simulink model "Online_Ordering_System_Activity_Diagram"  (R2024a)
settings: Solver=VariableStepAuto  StartTime=0.0  StopTime=10.0  RelTol=1e-3
(part 1 of 2)
settings Model: Creator=OdaNobuyuki  LastModifiedBy=OdaNobuyuki

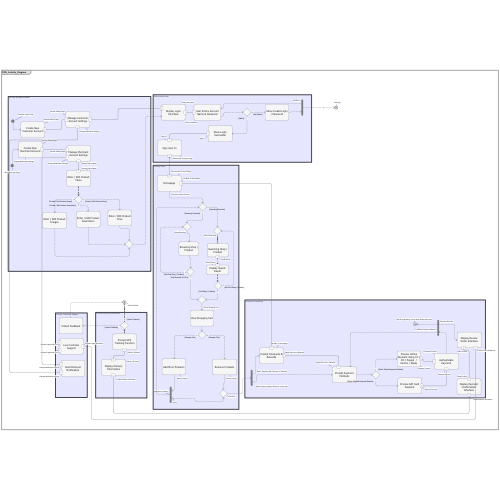
[thumbnail: Simulink's stored preview of the top-level diagram]
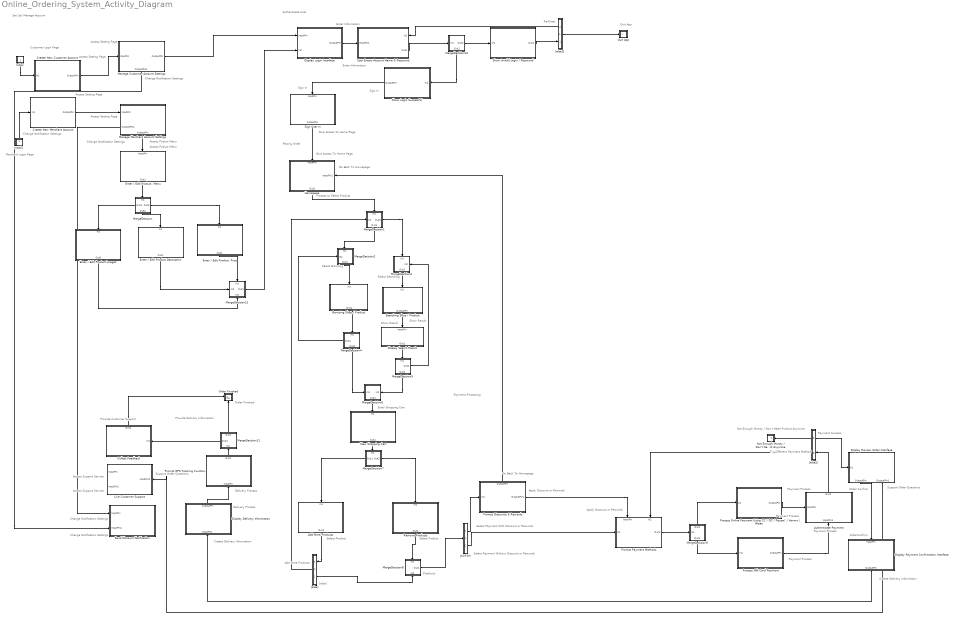
== system Online_Ordering_System_Activity_Diagram ==
  note: Support Order Questions
  note: Access Setting Page
  note: Re-Enter
  note: Enter Information
  note: Enter Information
  note: Give Access To Home Page
  note: Give Access To Home Page
  note: Show Result
  note: Show Result
  note: Access Support Service
  note: Change Notification Settings
  note: Change Notification Settings
  note: Change Notification Settings
  note: Provide Customer Support
  note: Merchant Login Page
  note: Customer Login Page
  note: Set Up/ Manage Account
  note: Delivery Process
  note: Delivery Process
  note: Create Delivery Information
  note: Create Delivery Information
  note: OrderConfirm
  note: Order Confirm
  note: Payment Success
  note: Try Different Payment Method
  note: Payment Process
  note: Payment Process
  note: Order Finished
  note: Quit App
  note: Not Enough Money / Don't Need Product Anymore
  note: Go Back To Homepage
  note: Apply Discount or Rewords
  note: Select Payment With Discount or Rewords
  note: Select Payment Without Discount or Rewords
  note: Enter Shopping Cart
  note: Add More Products
  note: Checkout
  note: [else]
  note: Select Product
  note: Select Product
  note: Select Searching
  note: Select Browsing
  note: Process to Select Product
  note: Sign In
  note: Provide Delivery Information
  note: Payment Processing
  note: Placing Order
  note: Authenticate User
  note: Access Setting Page
  note: Access Setting Page
  note: Access Setting Page
  note: Access Poduct Menu
  note: Access Poduct Menu
  note: Go Back To Homepage
  note: Apply Discount or Rewords
  note: Payment Process
  note: Payment Process
  note: Sign In
  note: Access Support Service
  note: Change Notification Settings
  note: Change Notification Settings
  note: Support Order Questions
  Add More Products : Subsystem
      settings: CopyFcn=set_param(gcbh,'LinkStatus','none');  PortSchema="{\"entries\":[{\"content\":{\"sides\":[{\"content\":{},\"type\":\"ConnectorPlacement.EquallySpacedRectSide\",\"uuid\":\"bfcd81ca-6cc0-42fb-99a3-45b9e2418847\"},{\"content\":{\"side\":\"RIGHT\"},\"type\":\"ConnectorPlacement.EquallySpacedRectSide\",\"uuid\":\"2a8794f4-3879-4bca-94c5-223b002e6000\"},{\"content\":{\"connectorIds\":[\"In1\"],\"side\":\"TOP\"},\"type\":\"ConnectorPlacement.EquallySpacedRectSide\",\"uuid\":\"3a486ab2-570b-44bd-b64c-1f33147c21a8\"},{\"content\":{\"connectorIds\":[\"Out1\"],\"side\":\"BOTTOM\"},\"type\":\"ConnectorPlacement.EquallySpacedRectSide\",\"uuid\":\"d015d86f-4011-41b5-baf2-3a54511849a1\"}]},\"type\":\"ConnectorPlacement.EquallySpacedConnector\",\"uuid\":\"4fcb30da-47fd-4892-8b00-93a0afe24f69\"}],\"packageUris\":[\"http://schema.mathworks.com/mf0/Connector/R2020b\"],\"version\":\"1.0\"}"
  Authenticate Payment : Subsystem
      settings: CopyFcn=set_param(gcbh,'LinkStatus','none');  PortSchema="{\"entries\":[{\"content\":{\"sides\":[{\"content\":{\"connectorIds\":[\"In1\"]},\"type\":\"ConnectorPlacement.EquallySpacedRectSide\",\"uuid\":\"be42d590-71f1-4328-bf36-769bf487d98c\"},{\"content\":{\"side\":\"RIGHT\"},\"type\":\"ConnectorPlacement.EquallySpacedRectSide\",\"uuid\":\"f686bdea-c754-42dd-9eaf-f93e30a31542\"},{\"content\":{\"connectorIds\":[\"Out1\"],\"side\":\"TOP\"},\"type\":\"ConnectorPlacement.EquallySpacedRectSide\",\"uuid\":\"aaf7fed9-1a14-44f9-b7af-ebaa0b7204d4\"},{\"content\":{\"connectorIds\":[\"In2\"],\"side\":\"BOTTOM\"},\"type\":\"ConnectorPlacement.EquallySpacedRectSide\",\"uuid\":\"9a6b8873-b7d5-47b2-be69-ed4b1ca685af\"}]},\"type\":\"ConnectorPlacement.EquallySpacedConnector\",\"uuid\":\"f2ca7d40-436a-4bcc-bce4-1a0ffaec5aa3\"}],\"packageUris\":[\"http://schema.mathworks.com/mf0/Connector/R2020b\"],\"version\":\"1.0\"}"
  Browsing Shop / Product : Subsystem
      settings: CopyFcn=set_param(gcbh,'LinkStatus','none');  PortSchema="{\"entries\":[{\"content\":{\"sides\":[{\"content\":{},\"type\":\"ConnectorPlacement.EquallySpacedRectSide\",\"uuid\":\"bfcd81ca-6cc0-42fb-99a3-45b9e2418847\"},{\"content\":{\"side\":\"RIGHT\"},\"type\":\"ConnectorPlacement.EquallySpacedRectSide\",\"uuid\":\"2a8794f4-3879-4bca-94c5-223b002e6000\"},{\"content\":{\"connectorIds\":[\"In1\"],\"side\":\"TOP\"},\"type\":\"ConnectorPlacement.EquallySpacedRectSide\",\"uuid\":\"3a486ab2-570b-44bd-b64c-1f33147c21a8\"},{\"content\":{\"connectorIds\":[\"Out1\"],\"side\":\"BOTTOM\"},\"type\":\"ConnectorPlacement.EquallySpacedRectSide\",\"uuid\":\"3ce360b7-2dac-440f-b63d-3367f7e15e3d\"}]},\"type\":\"ConnectorPlacement.EquallySpacedConnector\",\"uuid\":\"4fcb30da-47fd-4892-8b00-93a0afe24f69\"}],\"packageUris\":[\"http://schema.mathworks.com/mf0/Connector/R2020b\"],\"version\":\"1.0\"}"
  Collect Feedback : Subsystem
      settings: CopyFcn=set_param(gcbh,'LinkStatus','none');  PortSchema="{\"entries\":[{\"content\":{\"sides\":[{\"content\":{},\"type\":\"ConnectorPlacement.EquallySpacedRectSide\",\"uuid\":\"bfcd81ca-6cc0-42fb-99a3-45b9e2418847\"},{\"content\":{\"connectorIds\":[\"In1\"],\"side\":\"RIGHT\"},\"type\":\"ConnectorPlacement.EquallySpacedRectSide\",\"uuid\":\"2a8794f4-3879-4bca-94c5-223b002e6000\"},{\"content\":{\"connectorIds\":[\"Out1\"],\"side\":\"TOP\"},\"type\":\"ConnectorPlacement.EquallySpacedRectSide\",\"uuid\":\"3a486ab2-570b-44bd-b64c-1f33147c21a8\"}]},\"type\":\"ConnectorPlacement.EquallySpacedConnector\",\"uuid\":\"4fcb30da-47fd-4892-8b00-93a0afe24f69\"}],\"packageUris\":[\"http://schema.mathworks.com/mf0/Connector/R2020b\"],\"version\":\"1.0\"}"
  Create New Customer Account : Subsystem
      settings: CopyFcn=set_param(gcbh,'LinkStatus','none');
  Create New Merchant Account : Subsystem
      settings: CopyFcn=set_param(gcbh,'LinkStatus','none');
  Display Delivery Information : Subsystem
      settings: CopyFcn=set_param(gcbh,'LinkStatus','none');  PortSchema="{\"entries\":[{\"content\":{\"sides\":[{\"content\":{},\"type\":\"ConnectorPlacement.EquallySpacedRectSide\",\"uuid\":\"bfcd81ca-6cc0-42fb-99a3-45b9e2418847\"},{\"content\":{\"side\":\"RIGHT\"},\"type\":\"ConnectorPlacement.EquallySpacedRectSide\",\"uuid\":\"2a8794f4-3879-4bca-94c5-223b002e6000\"},{\"content\":{\"connectorIds\":[\"Out1\"],\"side\":\"TOP\"},\"type\":\"ConnectorPlacement.EquallySpacedRectSide\",\"uuid\":\"3a486ab2-570b-44bd-b64c-1f33147c21a8\"},{\"content\":{\"connectorIds\":[\"In1\"],\"side\":\"BOTTOM\"},\"type\":\"ConnectorPlacement.EquallySpacedRectSide\",\"uuid\":\"451f827c-7812-4a2b-baad-6237ef8a6df4\"}]},\"type\":\"ConnectorPlacement.EquallySpacedConnector\",\"uuid\":\"4fcb30da-47fd-4892-8b00-93a0afe24f69\"}],\"packageUris\":[\"http://schema.mathworks.com/mf0/Connector/R2020b\"],\"version\":\"1.0\"}"
  Display Login Interface : Subsystem
      settings: CopyFcn=set_param(gcbh,'LinkStatus','none');
  Display Payment Confirmation Interface : Subsystem
      settings: CopyFcn=set_param(gcbh,'LinkStatus','none');  PortSchema="{\"entries\":[{\"content\":{\"sides\":[{\"content\":{},\"type\":\"ConnectorPlacement.EquallySpacedRectSide\",\"uuid\":\"bfcd81ca-6cc0-42fb-99a3-45b9e2418847\"},{\"content\":{\"side\":\"RIGHT\"},\"type\":\"ConnectorPlacement.EquallySpacedRectSide\",\"uuid\":\"2a8794f4-3879-4bca-94c5-223b002e6000\"},{\"content\":{\"connectorIds\":[\"In1\"],\"side\":\"TOP\"},\"type\":\"ConnectorPlacement.EquallySpacedRectSide\",\"uuid\":\"3a486ab2-570b-44bd-b64c-1f33147c21a8\"},{\"content\":{\"connectorIds\":[\"Out1\"],\"side\":\"BOTTOM\"},\"type\":\"ConnectorPlacement.EquallySpacedRectSide\",\"uuid\":\"28139759-3bfc-43e8-9d7e-66a3114bf665\"}]},\"type\":\"ConnectorPlacement.EquallySpacedConnector\",\"uuid\":\"4fcb30da-47fd-4892-8b00-93a0afe24f69\"}],\"packageUris\":[\"http://schema.mathworks.com/mf0/Connector/R2020b\"],\"version\":\"1.0\"}"
  Display Review Order Interface : Subsystem
      settings: CopyFcn=set_param(gcbh,'LinkStatus','none');  PortSchema="{\"entries\":[{\"content\":{\"sides\":[{\"content\":{\"connectorIds\":[\"In1\"]},\"type\":\"ConnectorPlacement.EquallySpacedRectSide\",\"uuid\":\"6471ad79-39b4-4759-a736-ca09eeb8c1bf\"},{\"content\":{\"side\":\"RIGHT\"},\"type\":\"ConnectorPlacement.EquallySpacedRectSide\",\"uuid\":\"577ddd5b-f3b1-45a9-9feb-d7da88de3d28\"},{\"content\":{\"side\":\"TOP\"},\"type\":\"ConnectorPlacement.EquallySpacedRectSide\",\"uuid\":\"a229a248-5801-42c4-bc3a-df671f0dafbe\"},{\"content\":{\"connectorIds\":[\"Out1\",\"Out2\"],\"side\":\"BOTTOM\"},\"type\":\"ConnectorPlacement.EquallySpacedRectSide\",\"uuid\":\"31b6ee13-f671-41c4-9aa0-03afb235cf6a\"}]},\"type\":\"ConnectorPlacement.EquallySpacedConnector\",\"uuid\":\"7c76ea2b-17e6-4374-81ee-74665aad13d5\"}],\"packageUris\":[\"http://schema.mathworks.com/mf0/Connector/R2020b\"],\"version\":\"1.0\"}"
  Display Search Result : Subsystem
      settings: CopyFcn=set_param(gcbh,'LinkStatus','none');  PortSchema="{\"entries\":[{\"content\":{\"sides\":[{\"content\":{},\"type\":\"ConnectorPlacement.EquallySpacedRectSide\",\"uuid\":\"873ca6fb-737d-4b52-910b-d3362c79eeee\"},{\"content\":{\"side\":\"RIGHT\"},\"type\":\"ConnectorPlacement.EquallySpacedRectSide\",\"uuid\":\"ba60fc33-b236-4c23-8fcd-c0b31457fe6e\"},{\"content\":{\"connectorIds\":[\"In1\"],\"side\":\"TOP\"},\"type\":\"ConnectorPlacement.EquallySpacedRectSide\",\"uuid\":\"e81623ee-00f7-4aa0-b91b-b5c706a16c15\"},{\"content\":{\"connectorIds\":[\"Out1\"],\"side\":\"BOTTOM\"},\"type\":\"ConnectorPlacement.EquallySpacedRectSide\",\"uuid\":\"d2aa41e5-f0a2-4b95-961a-6292840acb60\"}]},\"type\":\"ConnectorPlacement.EquallySpacedConnector\",\"uuid\":\"4a5fb8e3-3bb7-4720-ba76-c4b22f03e2da\"}],\"packageUris\":[\"http://schema.mathworks.com/mf0/Connector/R2020b\"],\"version\":\"1.0\"}"
  Enter / Edit Product  Menu : Subsystem
      settings: CopyFcn=set_param(gcbh,'LinkStatus','none');  PortSchema="{\"entries\":[{\"content\":{\"sides\":[{\"content\":{},\"type\":\"ConnectorPlacement.EquallySpacedRectSide\",\"uuid\":\"873ca6fb-737d-4b52-910b-d3362c79eeee\"},{\"content\":{\"side\":\"RIGHT\"},\"type\":\"ConnectorPlacement.EquallySpacedRectSide\",\"uuid\":\"ba60fc33-b236-4c23-8fcd-c0b31457fe6e\"},{\"content\":{\"connectorIds\":[\"In1\"],\"side\":\"TOP\"},\"type\":\"ConnectorPlacement.EquallySpacedRectSide\",\"uuid\":\"e81623ee-00f7-4aa0-b91b-b5c706a16c15\"},{\"content\":{\"connectorIds\":[\"Out1\"],\"side\":\"BOTTOM\"},\"type\":\"ConnectorPlacement.EquallySpacedRectSide\",\"uuid\":\"f87e1b9f-2237-41b3-9347-c624be7169f3\"}]},\"type\":\"ConnectorPlacement.EquallySpacedConnector\",\"uuid\":\"4a5fb8e3-3bb7-4720-ba76-c4b22f03e2da\"}],\"packageUris\":[\"http://schema.mathworks.com/mf0/Connector/R2020b\"],\"version\":\"1.0\"}"
  Enter / Edit Product  Price : Subsystem
      settings: CopyFcn=set_param(gcbh,'LinkStatus','none');  PortSchema="{\"entries\":[{\"content\":{\"sides\":[{\"content\":{},\"type\":\"ConnectorPlacement.EquallySpacedRectSide\",\"uuid\":\"873ca6fb-737d-4b52-910b-d3362c79eeee\"},{\"content\":{\"side\":\"RIGHT\"},\"type\":\"ConnectorPlacement.EquallySpacedRectSide\",\"uuid\":\"ba60fc33-b236-4c23-8fcd-c0b31457fe6e\"},{\"content\":{\"connectorIds\":[\"In1\"],\"side\":\"TOP\"},\"type\":\"ConnectorPlacement.EquallySpacedRectSide\",\"uuid\":\"e81623ee-00f7-4aa0-b91b-b5c706a16c15\"},{\"content\":{\"connectorIds\":[\"Out1\"],\"side\":\"BOTTOM\"},\"type\":\"ConnectorPlacement.EquallySpacedRectSide\",\"uuid\":\"39b948d7-5fed-498d-a70d-5c860efeabd0\"}]},\"type\":\"ConnectorPlacement.EquallySpacedConnector\",\"uuid\":\"4a5fb8e3-3bb7-4720-ba76-c4b22f03e2da\"}],\"packageUris\":[\"http://schema.mathworks.com/mf0/Connector/R2020b\"],\"version\":\"1.0\"}"
  Enter / Edit Product Description : Subsystem
      settings: CopyFcn=set_param(gcbh,'LinkStatus','none');  PortSchema="{\"entries\":[{\"content\":{\"sides\":[{\"content\":{},\"type\":\"ConnectorPlacement.EquallySpacedRectSide\",\"uuid\":\"873ca6fb-737d-4b52-910b-d3362c79eeee\"},{\"content\":{\"side\":\"RIGHT\"},\"type\":\"ConnectorPlacement.EquallySpacedRectSide\",\"uuid\":\"ba60fc33-b236-4c23-8fcd-c0b31457fe6e\"},{\"content\":{\"connectorIds\":[\"In1\"],\"side\":\"TOP\"},\"type\":\"ConnectorPlacement.EquallySpacedRectSide\",\"uuid\":\"e81623ee-00f7-4aa0-b91b-b5c706a16c15\"},{\"content\":{\"connectorIds\":[\"Out1\"],\"side\":\"BOTTOM\"},\"type\":\"ConnectorPlacement.EquallySpacedRectSide\",\"uuid\":\"e9df8be3-2e0d-4814-bab8-e9195508b871\"}]},\"type\":\"ConnectorPlacement.EquallySpacedConnector\",\"uuid\":\"4a5fb8e3-3bb7-4720-ba76-c4b22f03e2da\"}],\"packageUris\":[\"http://schema.mathworks.com/mf0/Connector/R2020b\"],\"version\":\"1.0\"}"
  Enter / Edit Product Images : Subsystem
      settings: CopyFcn=set_param(gcbh,'LinkStatus','none');  PortSchema="{\"entries\":[{\"content\":{\"sides\":[{\"content\":{},\"type\":\"ConnectorPlacement.EquallySpacedRectSide\",\"uuid\":\"873ca6fb-737d-4b52-910b-d3362c79eeee\"},{\"content\":{\"side\":\"RIGHT\"},\"type\":\"ConnectorPlacement.EquallySpacedRectSide\",\"uuid\":\"ba60fc33-b236-4c23-8fcd-c0b31457fe6e\"},{\"content\":{\"connectorIds\":[\"In1\"],\"side\":\"TOP\"},\"type\":\"ConnectorPlacement.EquallySpacedRectSide\",\"uuid\":\"e81623ee-00f7-4aa0-b91b-b5c706a16c15\"},{\"content\":{\"connectorIds\":[\"Out1\"],\"side\":\"BOTTOM\"},\"type\":\"ConnectorPlacement.EquallySpacedRectSide\",\"uuid\":\"a34f8f4a-2331-4593-96e1-216def65723d\"}]},\"type\":\"ConnectorPlacement.EquallySpacedConnector\",\"uuid\":\"4a5fb8e3-3bb7-4720-ba76-c4b22f03e2da\"}],\"packageUris\":[\"http://schema.mathworks.com/mf0/Connector/R2020b\"],\"version\":\"1.0\"}"
  Homepage : Subsystem
      settings: CopyFcn=set_param(gcbh,'LinkStatus','none');  PortSchema="{\"entries\":[{\"content\":{\"sides\":[{\"content\":{},\"type\":\"ConnectorPlacement.EquallySpacedRectSide\",\"uuid\":\"9c7be66a-1772-4efc-8f14-7a500ca71a54\"},{\"content\":{\"connectorIds\":[\"In2\"],\"side\":\"RIGHT\"},\"type\":\"ConnectorPlacement.EquallySpacedRectSide\",\"uuid\":\"38f08e10-8633-45ed-b24d-07e293b2144f\"},{\"content\":{\"connectorIds\":[\"In1\"],\"side\":\"TOP\"},\"type\":\"ConnectorPlacement.EquallySpacedRectSide\",\"uuid\":\"9945d600-1a94-418c-9fd4-80c3bf52b6dd\"},{\"content\":{\"connectorIds\":[\"Out1\"],\"side\":\"BOTTOM\"},\"type\":\"ConnectorPlacement.EquallySpacedRectSide\",\"uuid\":\"639fe1aa-fc4f-4338-a28d-cf257359008e\"}]},\"type\":\"ConnectorPlacement.EquallySpacedConnector\",\"uuid\":\"f5f1796a-aeed-4e15-b522-4d9bae7d766e\"}],\"packageUris\":[\"http://schema.mathworks.com/mf0/Connector/R2020b\"],\"version\":\"1.0\"}"
  Initial : Subsystem
      settings: CopyFcn=set_param(gcbh,'LinkStatus','none');  PortSchema="{\"entries\":[{\"content\":{\"sides\":[{\"content\":{},\"type\":\"ConnectorPlacement.EquallySpacedRectSide\",\"uuid\":\"873ca6fb-737d-4b52-910b-d3362c79eeee\"},{\"content\":{\"side\":\"RIGHT\"},\"type\":\"ConnectorPlacement.EquallySpacedRectSide\",\"uuid\":\"ba60fc33-b236-4c23-8fcd-c0b31457fe6e\"},{\"content\":{\"side\":\"TOP\"},\"type\":\"ConnectorPlacement.EquallySpacedRectSide\",\"uuid\":\"e81623ee-00f7-4aa0-b91b-b5c706a16c15\"},{\"content\":{\"connectorIds\":[\"Out1\"],\"side\":\"BOTTOM\"},\"type\":\"ConnectorPlacement.EquallySpacedRectSide\",\"uuid\":\"754ea620-bcdd-4f6e-b1d6-7350cee697a7\"}]},\"type\":\"ConnectorPlacement.EquallySpacedConnector\",\"uuid\":\"4a5fb8e3-3bb7-4720-ba76-c4b22f03e2da\"}],\"packageUris\":[\"http://schema.mathworks.com/mf0/Connector/R2020b\"],\"version\":\"1.0\"}"
  Initial1 : Subsystem
      settings: CopyFcn=set_param(gcbh,'LinkStatus','none');  PortSchema="{\"entries\":[{\"content\":{\"sides\":[{\"content\":{},\"type\":\"ConnectorPlacement.EquallySpacedRectSide\",\"uuid\":\"873ca6fb-737d-4b52-910b-d3362c79eeee\"},{\"content\":{\"side\":\"RIGHT\"},\"type\":\"ConnectorPlacement.EquallySpacedRectSide\",\"uuid\":\"ba60fc33-b236-4c23-8fcd-c0b31457fe6e\"},{\"content\":{\"connectorIds\":[\"Out1\"],\"side\":\"TOP\"},\"type\":\"ConnectorPlacement.EquallySpacedRectSide\",\"uuid\":\"e81623ee-00f7-4aa0-b91b-b5c706a16c15\"}]},\"type\":\"ConnectorPlacement.EquallySpacedConnector\",\"uuid\":\"4a5fb8e3-3bb7-4720-ba76-c4b22f03e2da\"}],\"packageUris\":[\"http://schema.mathworks.com/mf0/Connector/R2020b\"],\"version\":\"1.0\"}"
  JoinFork : Subsystem
      settings: CopyFcn=set_param(gcbh,'LinkStatus','none');
  Live Customer Support : Subsystem
      settings: CopyFcn=set_param(gcbh,'LinkStatus','none');  PortSchema="{\"entries\":[{\"content\":{\"sides\":[{\"content\":{\"connectorIds\":[\"In1\",\"In2\"]},\"type\":\"ConnectorPlacement.EquallySpacedRectSide\",\"uuid\":\"5dac1142-e9ce-43d0-ba52-63279954a8b9\"},{\"content\":{\"connectorIds\":[\"In3\"],\"side\":\"RIGHT\"},\"type\":\"ConnectorPlacement.EquallySpacedRectSide\",\"uuid\":\"ca4fd33a-c89a-4006-bed6-b92bcf697d1b\"},{\"content\":{\"side\":\"TOP\"},\"type\":\"ConnectorPlacement.EquallySpacedRectSide\",\"uuid\":\"932f8a37-4771-496a-b31b-228ed95da92a\"}]},\"type\":\"ConnectorPlacement.EquallySpacedConnector\",\"uuid\":\"cf714b23-59d2-41ff-98fd-22561387faef\"}],\"packageUris\":[\"http://schema.mathworks.com/mf0/Connector/R2020b\"],\"version\":\"1.0\"}"
  Manage Customer Account Settings : Subsystem
      settings: CopyFcn=set_param(gcbh,'LinkStatus','none');  PortSchema="{\"entries\":[{\"content\":{\"sides\":[{\"content\":{\"connectorIds\":[\"In1\"]},\"type\":\"ConnectorPlacement.EquallySpacedRectSide\",\"uuid\":\"3fb5762c-1463-4d69-b71f-d3478a8e66fc\"},{\"content\":{\"connectorIds\":[\"Out1\"],\"side\":\"RIGHT\"},\"type\":\"ConnectorPlacement.EquallySpacedRectSide\",\"uuid\":\"8c5ab484-2882-4a25-a56e-8782928f7c87\"},{\"content\":{\"side\":\"TOP\"},\"type\":\"ConnectorPlacement.EquallySpacedRectSide\",\"uuid\":\"adc29f19-0a83-4db7-81d6-093442179a8b\"},{\"content\":{\"connectorIds\":[\"Out2\"],\"side\":\"BOTTOM\"},\"type\":\"ConnectorPlacement.EquallySpacedRectSide\",\"uuid\":\"551acee2-b4f2-469f-bccf-f435c30cc1a3\"}]},\"type\":\"ConnectorPlacement.EquallySpacedConnector\",\"uuid\":\"53417cf2-4b18-460a-8f45-b9110c6542e4\"}],\"packageUris\":[\"http://schema.mathworks.com/mf0/Connector/R2020b\"],\"version\":\"1.0\"}"
  Manage Merchant Account Settings : Subsystem
      settings: CopyFcn=set_param(gcbh,'LinkStatus','none');  PortSchema="{\"entries\":[{\"content\":{\"sides\":[{\"content\":{\"connectorIds\":[\"In1\",\"Out2\"]},\"type\":\"ConnectorPlacement.EquallySpacedRectSide\",\"uuid\":\"be42d590-71f1-4328-bf36-769bf487d98c\"},{\"content\":{\"side\":\"RIGHT\"},\"type\":\"ConnectorPlacement.EquallySpacedRectSide\",\"uuid\":\"f686bdea-c754-42dd-9eaf-f93e30a31542\"},{\"content\":{\"side\":\"TOP\"},\"type\":\"ConnectorPlacement.EquallySpacedRectSide\",\"uuid\":\"aaf7fed9-1a14-44f9-b7af-ebaa0b7204d4\"},{\"content\":{\"connectorIds\":[\"Out1\"],\"side\":\"BOTTOM\"},\"type\":\"ConnectorPlacement.EquallySpacedRectSide\",\"uuid\":\"0a28ab33-b43c-4e05-97e4-fa4d8c4772ab\"}]},\"type\":\"ConnectorPlacement.EquallySpacedConnector\",\"uuid\":\"f2ca7d40-436a-4bcc-bce4-1a0ffaec5aa3\"}],\"packageUris\":[\"http://schema.mathworks.com/mf0/Connector/R2020b\"],\"version\":\"1.0\"}"
  MergeDecision : Subsystem
      settings: CopyFcn=set_param(gcbh,'LinkStatus','none');  PortSchema="{\"entries\":[{\"content\":{\"sides\":[{\"content\":{\"connectorIds\":[\"Out3\"]},\"type\":\"ConnectorPlacement.EquallySpacedRectSide\",\"uuid\":\"873ca6fb-737d-4b52-910b-d3362c79eeee\"},{\"content\":{\"connectorIds\":[\"Out1\"],\"side\":\"RIGHT\"},\"type\":\"ConnectorPlacement.EquallySpacedRectSide\",\"uuid\":\"ba60fc33-b236-4c23-8fcd-c0b31457fe6e\"},{\"content\":{\"connectorIds\":[\"In1\"],\"side\":\"TOP\"},\"type\":\"ConnectorPlacement.EquallySpacedRectSide\",\"uuid\":\"e81623ee-00f7-4aa0-b91b-b5c706a16c15\"},{\"content\":{\"connectorIds\":[\"Out2\"],\"side\":\"BOTTOM\"},\"type\":\"ConnectorPlacement.EquallySpacedRectSide\",\"uuid\":\"502fd812-fb61-4656-820a-d2df7cf81d1a\"}]},\"type\":\"ConnectorPlacement.EquallySpacedConnector\",\"uuid\":\"4a5fb8e3-3bb7-4720-ba76-c4b22f03e2da\"}],\"packageUris\":[\"http://schema.mathworks.com/mf0/Connector/R2020b\"],\"version\":\"1.0\"}"
  MergeDecision1 : Subsystem
      settings: CopyFcn=set_param(gcbh,'LinkStatus','none');  PortSchema="{\"entries\":[{\"content\":{\"sides\":[{\"content\":{\"connectorIds\":[\"In1\"]},\"type\":\"ConnectorPlacement.EquallySpacedRectSide\",\"uuid\":\"bfcd81ca-6cc0-42fb-99a3-45b9e2418847\"},{\"content\":{\"connectorIds\":[\"Out1\"],\"side\":\"RIGHT\"},\"type\":\"ConnectorPlacement.EquallySpacedRectSide\",\"uuid\":\"2a8794f4-3879-4bca-94c5-223b002e6000\"},{\"content\":{\"connectorIds\":[\"In2\"],\"side\":\"TOP\"},\"type\":\"ConnectorPlacement.EquallySpacedRectSide\",\"uuid\":\"3a486ab2-570b-44bd-b64c-1f33147c21a8\"},{\"content\":{\"connectorIds\":[\"Out2\"],\"side\":\"BOTTOM\"},\"type\":\"ConnectorPlacement.EquallySpacedRectSide\",\"uuid\":\"dfbb0019-e897-4582-8c2c-93c64ac312f3\"}]},\"type\":\"ConnectorPlacement.EquallySpacedConnector\",\"uuid\":\"4fcb30da-47fd-4892-8b00-93a0afe24f69\"}],\"packageUris\":[\"http://schema.mathworks.com/mf0/Connector/R2020b\"],\"version\":\"1.0\"}"
  MergeDecision10 : Subsystem
      settings: CopyFcn=set_param(gcbh,'LinkStatus','none');  PortSchema="{\"entries\":[{\"content\":{\"sides\":[{\"content\":{\"connectorIds\":[\"In1\"]},\"type\":\"ConnectorPlacement.EquallySpacedRectSide\",\"uuid\":\"be42d590-71f1-4328-bf36-769bf487d98c\"},{\"content\":{\"connectorIds\":[\"Out1\"],\"side\":\"RIGHT\"},\"type\":\"ConnectorPlacement.EquallySpacedRectSide\",\"uuid\":\"f686bdea-c754-42dd-9eaf-f93e30a31542\"},{\"content\":{\"side\":\"TOP\"},\"type\":\"ConnectorPlacement.EquallySpacedRectSide\",\"uuid\":\"aaf7fed9-1a14-44f9-b7af-ebaa0b7204d4\"},{\"content\":{\"connectorIds\":[\"Out2\"],\"side\":\"BOTTOM\"},\"type\":\"ConnectorPlacement.EquallySpacedRectSide\",\"uuid\":\"1f81f839-6f9d-4f3b-a3c4-dc8895f723be\"}]},\"type\":\"ConnectorPlacement.EquallySpacedConnector\",\"uuid\":\"f2ca7d40-436a-4bcc-bce4-1a0ffaec5aa3\"}],\"packageUris\":[\"http://schema.mathworks.com/mf0/Connector/R2020b\"],\"version\":\"1.0\"}"
  MergeDecision11 : Subsystem
      settings: CopyFcn=set_param(gcbh,'LinkStatus','none');  PortSchema="{\"entries\":[{\"content\":{\"sides\":[{\"content\":{\"connectorIds\":[\"Out2\"]},\"type\":\"ConnectorPlacement.EquallySpacedRectSide\",\"uuid\":\"bfcd81ca-6cc0-42fb-99a3-45b9e2418847\"},{\"content\":{\"side\":\"RIGHT\"},\"type\":\"ConnectorPlacement.EquallySpacedRectSide\",\"uuid\":\"2a8794f4-3879-4bca-94c5-223b002e6000\"},{\"content\":{\"connectorIds\":[\"Out1\"],\"side\":\"TOP\"},\"type\":\"ConnectorPlacement.EquallySpacedRectSide\",\"uuid\":\"3a486ab2-570b-44bd-b64c-1f33147c21a8\"},{\"content\":{\"connectorIds\":[\"In1\"],\"side\":\"BOTTOM\"},\"type\":\"ConnectorPlacement.EquallySpacedRectSide\",\"uuid\":\"55917b43-766e-45bf-9655-6aa6f34d9f1e\"}]},\"type\":\"ConnectorPlacement.EquallySpacedConnector\",\"uuid\":\"4fcb30da-47fd-4892-8b00-93a0afe24f69\"}],\"packageUris\":[\"http://schema.mathworks.com/mf0/Connector/R2020b\"],\"version\":\"1.0\"}"
  MergeDecision12 : Subsystem
      settings: CopyFcn=set_param(gcbh,'LinkStatus','none');  PortSchema="{\"entries\":[{\"content\":{\"sides\":[{\"content\":{\"connectorIds\":[\"In1\"]},\"type\":\"ConnectorPlacement.EquallySpacedRectSide\",\"uuid\":\"b6348e20-82e8-4a77-8276-f517ac215c0d\"},{\"content\":{\"connectorIds\":[\"Out1\"],\"side\":\"RIGHT\"},\"type\":\"ConnectorPlacement.EquallySpacedRectSide\",\"uuid\":\"e8bfeca0-0d80-4710-8b22-b5779b08de1c\"},{\"content\":{\"connectorIds\":[\"In2\"],\"side\":\"TOP\"},\"type\":\"ConnectorPlacement.EquallySpacedRectSide\",\"uuid\":\"c80e6f29-4c6c-40d0-ba69-4682bae4d315\"},{\"content\":{\"connectorIds\":[\"In3\"],\"side\":\"BOTTOM\"},\"type\":\"ConnectorPlacement.EquallySpacedRectSide\",\"uuid\":\"618f9ff1-83d9-4ba7-b824-91f6f00ab0ec\"}]},\"type\":\"ConnectorPlacement.EquallySpacedConnector\",\"uuid\":\"787878f5-e7c0-4999-b8b1-5d654517abb5\"}],\"packageUris\":[\"http://schema.mathworks.com/mf0/Connector/R2020b\"],\"version\":\"1.0\"}"
  MergeDecision2 : Subsystem
      settings: CopyFcn=set_param(gcbh,'LinkStatus','none');  PortSchema="{\"entries\":[{\"content\":{\"sides\":[{\"content\":{\"connectorIds\":[\"In1\"]},\"type\":\"ConnectorPlacement.EquallySpacedRectSide\",\"uuid\":\"bfcd81ca-6cc0-42fb-99a3-45b9e2418847\"},{\"content\":{\"side\":\"RIGHT\"},\"type\":\"ConnectorPlacement.EquallySpacedRectSide\",\"uuid\":\"2a8794f4-3879-4bca-94c5-223b002e6000\"},{\"content\":{\"connectorIds\":[\"In2\"],\"side\":\"TOP\"},\"type\":\"ConnectorPlacement.EquallySpacedRectSide\",\"uuid\":\"3a486ab2-570b-44bd-b64c-1f33147c21a8\"},{\"content\":{\"connectorIds\":[\"Out1\"],\"side\":\"BOTTOM\"},\"type\":\"ConnectorPlacement.EquallySpacedRectSide\",\"uuid\":\"2b514eea-2618-4277-9ff0-bc9e5342f5b1\"}]},\"type\":\"ConnectorPlacement.EquallySpacedConnector\",\"uuid\":\"4fcb30da-47fd-4892-8b00-93a0afe24f69\"}],\"packageUris\":[\"http://schema.mathworks.com/mf0/Connector/R2020b\"],\"version\":\"1.0\"}"
  MergeDecision3 : Subsystem
      settings: CopyFcn=set_param(gcbh,'LinkStatus','none');  PortSchema="{\"entries\":[{\"content\":{\"sides\":[{\"content\":{},\"type\":\"ConnectorPlacement.EquallySpacedRectSide\",\"uuid\":\"bfcd81ca-6cc0-42fb-99a3-45b9e2418847\"},{\"content\":{\"connectorIds\":[\"In2\"],\"side\":\"RIGHT\"},\"type\":\"ConnectorPlacement.EquallySpacedRectSide\",\"uuid\":\"2a8794f4-3879-4bca-94c5-223b002e6000\"},{\"content\":{\"connectorIds\":[\"In1\"],\"side\":\"TOP\"},\"type\":\"ConnectorPlacement.EquallySpacedRectSide\",\"uuid\":\"3a486ab2-570b-44bd-b64c-1f33147c21a8\"},{\"content\":{\"connectorIds\":[\"Out1\"],\"side\":\"BOTTOM\"},\"type\":\"ConnectorPlacement.EquallySpacedRectSide\",\"uuid\":\"c2f41a78-1dbb-4966-aa89-36c67e16d6e6\"}]},\"type\":\"ConnectorPlacement.EquallySpacedConnector\",\"uuid\":\"4fcb30da-47fd-4892-8b00-93a0afe24f69\"}],\"packageUris\":[\"http://schema.mathworks.com/mf0/Connector/R2020b\"],\"version\":\"1.0\"}"
  MergeDecision4 : Subsystem
      settings: CopyFcn=set_param(gcbh,'LinkStatus','none');  PortSchema="{\"entries\":[{\"content\":{\"sides\":[{\"content\":{\"connectorIds\":[\"Out2\"]},\"type\":\"ConnectorPlacement.EquallySpacedRectSide\",\"uuid\":\"bfcd81ca-6cc0-42fb-99a3-45b9e2418847\"},{\"content\":{\"side\":\"RIGHT\"},\"type\":\"ConnectorPlacement.EquallySpacedRectSide\",\"uuid\":\"2a8794f4-3879-4bca-94c5-223b002e6000\"},{\"content\":{\"connectorIds\":[\"In1\"],\"side\":\"TOP\"},\"type\":\"ConnectorPlacement.EquallySpacedRectSide\",\"uuid\":\"3a486ab2-570b-44bd-b64c-1f33147c21a8\"},{\"content\":{\"connectorIds\":[\"Out1\"],\"side\":\"BOTTOM\"},\"type\":\"ConnectorPlacement.EquallySpacedRectSide\",\"uuid\":\"008cc571-7a64-41c4-a992-12556a9e9460\"}]},\"type\":\"ConnectorPlacement.EquallySpacedConnector\",\"uuid\":\"4fcb30da-47fd-4892-8b00-93a0afe24f69\"}],\"packageUris\":[\"http://schema.mathworks.com/mf0/Connector/R2020b\"],\"version\":\"1.0\"}"
  MergeDecision5 : Subsystem
      settings: CopyFcn=set_param(gcbh,'LinkStatus','none');  PortSchema="{\"entries\":[{\"content\":{\"sides\":[{\"content\":{},\"type\":\"ConnectorPlacement.EquallySpacedRectSide\",\"uuid\":\"bfcd81ca-6cc0-42fb-99a3-45b9e2418847\"},{\"content\":{\"connectorIds\":[\"Out1\"],\"side\":\"RIGHT\"},\"type\":\"ConnectorPlacement.EquallySpacedRectSide\",\"uuid\":\"2a8794f4-3879-4bca-94c5-223b002e6000\"},{\"content\":{\"connectorIds\":[\"In1\"],\"side\":\"TOP\"},\"type\":\"ConnectorPlacement.EquallySpacedRectSide\",\"uuid\":\"3a486ab2-570b-44bd-b64c-1f33147c21a8\"},{\"content\":{\"connectorIds\":[\"Out2\"],\"side\":\"BOTTOM\"},\"type\":\"ConnectorPlacement.EquallySpacedRectSide\",\"uuid\":\"d88ca2bd-bba1-45f0-87d6-11369fc701db\"}]},\"type\":\"ConnectorPlacement.EquallySpacedConnector\",\"uuid\":\"4fcb30da-47fd-4892-8b00-93a0afe24f69\"}],\"packageUris\":[\"http://schema.mathworks.com/mf0/Connector/R2020b\"],\"version\":\"1.0\"}"
  MergeDecision6 : Subsystem
      settings: CopyFcn=set_param(gcbh,'LinkStatus','none');  PortSchema="{\"entries\":[{\"content\":{\"sides\":[{\"content\":{\"connectorIds\":[\"In1\"]},\"type\":\"ConnectorPlacement.EquallySpacedRectSide\",\"uuid\":\"6471ad79-39b4-4759-a736-ca09eeb8c1bf\"},{\"content\":{\"connectorIds\":[\"In2\"],\"side\":\"RIGHT\"},\"type\":\"ConnectorPlacement.EquallySpacedRectSide\",\"uuid\":\"577ddd5b-f3b1-45a9-9feb-d7da88de3d28\"},{\"content\":{\"side\":\"TOP\"},\"type\":\"ConnectorPlacement.EquallySpacedRectSide\",\"uuid\":\"a229a248-5801-42c4-bc3a-df671f0dafbe\"},{\"content\":{\"connectorIds\":[\"Out1\"],\"side\":\"BOTTOM\"},\"type\":\"ConnectorPlacement.EquallySpacedRectSide\",\"uuid\":\"311dc0cd-b161-4cfb-8bab-773e5f746b42\"}]},\"type\":\"ConnectorPlacement.EquallySpacedConnector\",\"uuid\":\"7c76ea2b-17e6-4374-81ee-74665aad13d5\"}],\"packageUris\":[\"http://schema.mathworks.com/mf0/Connector/R2020b\"],\"version\":\"1.0\"}"
  MergeDecision7 : Subsystem
      settings: CopyFcn=set_param(gcbh,'LinkStatus','none');  PortSchema="{\"entries\":[{\"content\":{\"sides\":[{\"content\":{\"connectorIds\":[\"Out2\"]},\"type\":\"ConnectorPlacement.EquallySpacedRectSide\",\"uuid\":\"bfcd81ca-6cc0-42fb-99a3-45b9e2418847\"},{\"content\":{\"connectorIds\":[\"Out1\"],\"side\":\"RIGHT\"},\"type\":\"ConnectorPlacement.EquallySpacedRectSide\",\"uuid\":\"2a8794f4-3879-4bca-94c5-223b002e6000\"},{\"content\":{\"connectorIds\":[\"In1\"],\"side\":\"TOP\"},\"type\":\"ConnectorPlacement.EquallySpacedRectSide\",\"uuid\":\"3a486ab2-570b-44bd-b64c-1f33147c21a8\"}]},\"type\":\"ConnectorPlacement.EquallySpacedConnector\",\"uuid\":\"4fcb30da-47fd-4892-8b00-93a0afe24f69\"}],\"packageUris\":[\"http://schema.mathworks.com/mf0/Connector/R2020b\"],\"version\":\"1.0\"}"
  MergeDecision8 : Subsystem
      settings: CopyFcn=set_param(gcbh,'LinkStatus','none');  PortSchema="{\"entries\":[{\"content\":{\"sides\":[{\"content\":{},\"type\":\"ConnectorPlacement.EquallySpacedRectSide\",\"uuid\":\"bfcd81ca-6cc0-42fb-99a3-45b9e2418847\"},{\"content\":{\"connectorIds\":[\"Out1\"],\"side\":\"RIGHT\"},\"type\":\"ConnectorPlacement.EquallySpacedRectSide\",\"uuid\":\"2a8794f4-3879-4bca-94c5-223b002e6000\"},{\"content\":{\"connectorIds\":[\"In1\"],\"side\":\"TOP\"},\"type\":\"ConnectorPlacement.EquallySpacedRectSide\",\"uuid\":\"3a486ab2-570b-44bd-b64c-1f33147c21a8\"},{\"content\":{\"connectorIds\":[\"In2\"],\"side\":\"BOTTOM\"},\"type\":\"ConnectorPlacement.EquallySpacedRectSide\",\"uuid\":\"0cf9ed2b-e2ff-4baf-8dc3-4873fb6f6a87\"}]},\"type\":\"ConnectorPlacement.EquallySpacedConnector\",\"uuid\":\"4fcb30da-47fd-4892-8b00-93a0afe24f69\"}],\"packageUris\":[\"http://schema.mathworks.com/mf0/Connector/R2020b\"],\"version\":\"1.0\"}"
  MergeDecision9 : Subsystem
      settings: CopyFcn=set_param(gcbh,'LinkStatus','none');  PortSchema="{\"entries\":[{\"content\":{\"sides\":[{\"content\":{\"connectorIds\":[\"In1\"]},\"type\":\"ConnectorPlacement.EquallySpacedRectSide\",\"uuid\":\"bfcd81ca-6cc0-42fb-99a3-45b9e2418847\"},{\"content\":{\"side\":\"RIGHT\"},\"type\":\"ConnectorPlacement.EquallySpacedRectSide\",\"uuid\":\"2a8794f4-3879-4bca-94c5-223b002e6000\"},{\"content\":{\"connectorIds\":[\"Out2\"],\"side\":\"TOP\"},\"type\":\"ConnectorPlacement.EquallySpacedRectSide\",\"uuid\":\"3a486ab2-570b-44bd-b64c-1f33147c21a8\"},{\"content\":{\"connectorIds\":[\"Out1\"],\"side\":\"BOTTOM\"},\"type\":\"ConnectorPlacement.EquallySpacedRectSide\",\"uuid\":\"4a841506-082d-4ac6-9900-2ff85b03c56a\"}]},\"type\":\"ConnectorPlacement.EquallySpacedConnector\",\"uuid\":\"4fcb30da-47fd-4892-8b00-93a0afe24f69\"}],\"packageUris\":[\"http://schema.mathworks.com/mf0/Connector/R2020b\"],\"version\":\"1.0\"}"
  Not Enough Money / Don't Need Product Anymore : Subsystem
      settings: CopyFcn=set_param(gcbh,'LinkStatus','none');  PortSchema="{\"entries\":[{\"content\":{\"sides\":[{\"content\":{},\"type\":\"ConnectorPlacement.EquallySpacedRectSide\",\"uuid\":\"bfcd81ca-6cc0-42fb-99a3-45b9e2418847\"},{\"content\":{\"connectorIds\":[\"In1\"],\"side\":\"RIGHT\"},\"type\":\"ConnectorPlacement.EquallySpacedRectSide\",\"uuid\":\"2a8794f4-3879-4bca-94c5-223b002e6000\"},{\"content\":{\"side\":\"TOP\"},\"type\":\"ConnectorPlacement.EquallySpacedRectSide\",\"uuid\":\"3a486ab2-570b-44bd-b64c-1f33147c21a8\"},{\"content\":{\"side\":\"BOTTOM\"},\"type\":\"ConnectorPlacement.EquallySpacedRectSide\",\"uuid\":\"b8e02093-9ac8-40bd-8ea2-34c667592cca\"}]},\"type\":\"ConnectorPlacement.EquallySpacedConnector\",\"uuid\":\"4fcb30da-47fd-4892-8b00-93a0afe24f69\"}],\"packageUris\":[\"http://schema.mathworks.com/mf0/Connector/R2020b\"],\"version\":\"1.0\"}"
  Order Finished : Subsystem
      settings: CopyFcn=set_param(gcbh,'LinkStatus','none');  PortSchema="{\"entries\":[{\"content\":{\"sides\":[{\"content\":{\"connectorIds\":[\"In1\"]},\"type\":\"ConnectorPlacement.EquallySpacedRectSide\",\"uuid\":\"bfcd81ca-6cc0-42fb-99a3-45b9e2418847\"},{\"content\":{\"side\":\"RIGHT\"},\"type\":\"ConnectorPlacement.EquallySpacedRectSide\",\"uuid\":\"2a8794f4-3879-4bca-94c5-223b002e6000\"},{\"content\":{\"side\":\"TOP\"},\"type\":\"ConnectorPlacement.EquallySpacedRectSide\",\"uuid\":\"3a486ab2-570b-44bd-b64c-1f33147c21a8\"},{\"content\":{\"connectorIds\":[\"In2\"],\"side\":\"BOTTOM\"},\"type\":\"ConnectorPlacement.EquallySpacedRectSide\",\"uuid\":\"f6c49d25-dc2c-4642-870d-3e0b1c73bf64\"}]},\"type\":\"ConnectorPlacement.EquallySpacedConnector\",\"uuid\":\"4fcb30da-47fd-4892-8b00-93a0afe24f69\"}],\"packageUris\":[\"http://schema.mathworks.com/mf0/Connector/R2020b\"],\"version\":\"1.0\"}"
  Process Gift Card Payment : Subsystem
      settings: CopyFcn=set_param(gcbh,'LinkStatus','none');
  Process Online Payment Using CC / DC / Paypal  / Venmo / Alipay : Subsystem
      settings: CopyFcn=set_param(gcbh,'LinkStatus','none');
  Prompt Discounts & Rewords : Subsystem
      settings: CopyFcn=set_param(gcbh,'LinkStatus','none');  PortSchema="{\"entries\":[{\"content\":{\"sides\":[{\"content\":{\"connectorIds\":[\"In1\"]},\"type\":\"ConnectorPlacement.EquallySpacedRectSide\",\"uuid\":\"698359e7-1191-4a0c-9b28-01ff2ab516cf\"},{\"content\":{\"connectorIds\":[\"Out1\"],\"side\":\"RIGHT\"},\"type\":\"ConnectorPlacement.EquallySpacedRectSide\",\"uuid\":\"4ad4a9c2-faf3-4004-ab2d-af7e32192da7\"},{\"content\":{\"connectorIds\":[\"Out2\"],\"side\":\"TOP\"},\"type\":\"ConnectorPlacement.EquallySpacedRectSide\",\"uuid\":\"96e906c2-c001-46b7-b0f9-08edb441f529\"}]},\"type\":\"ConnectorPlacement.EquallySpacedConnector\",\"uuid\":\"b69dc501-630f-4122-b2c0-bba745382e91\"}],\"packageUris\":[\"http://schema.mathworks.com/mf0/Connector/R2020b\"],\"version\":\"1.0\"}"
  Prompt GPS Tracking Function : Subsystem
      settings: CopyFcn=set_param(gcbh,'LinkStatus','none');  PortSchema="{\"entries\":[{\"content\":{\"sides\":[{\"content\":{},\"type\":\"ConnectorPlacement.EquallySpacedRectSide\",\"uuid\":\"bfcd81ca-6cc0-42fb-99a3-45b9e2418847\"},{\"content\":{\"side\":\"RIGHT\"},\"type\":\"ConnectorPlacement.EquallySpacedRectSide\",\"uuid\":\"2a8794f4-3879-4bca-94c5-223b002e6000\"},{\"content\":{\"connectorIds\":[\"Out1\"],\"side\":\"TOP\"},\"type\":\"ConnectorPlacement.EquallySpacedRectSide\",\"uuid\":\"3a486ab2-570b-44bd-b64c-1f33147c21a8\"},{\"content\":{\"connectorIds\":[\"In1\"],\"side\":\"BOTTOM\"},\"type\":\"ConnectorPlacement.EquallySpacedRectSide\",\"uuid\":\"cbf92014-a959-4db7-a22c-6767a3efb1c3\"}]},\"type\":\"ConnectorPlacement.EquallySpacedConnector\",\"uuid\":\"4fcb30da-47fd-4892-8b00-93a0afe24f69\"}],\"packageUris\":[\"http://schema.mathworks.com/mf0/Connector/R2020b\"],\"version\":\"1.0\"}"
  Prompt Payment Methods : Subsystem
      settings: CopyFcn=set_param(gcbh,'LinkStatus','none');  PortSchema="{\"entries\":[{\"content\":{\"sides\":[{\"content\":{\"connectorIds\":[\"In1\"]},\"type\":\"ConnectorPlacement.EquallySpacedRectSide\",\"uuid\":\"628b8bbf-248c-40ae-9019-a4b7410bd852\"},{\"content\":{\"connectorIds\":[\"Out1\"],\"side\":\"RIGHT\"},\"type\":\"ConnectorPlacement.EquallySpacedRectSide\",\"uuid\":\"6f0a6d2f-3917-4433-a509-63fc1b11366d\"},{\"content\":{\"connectorIds\":[\"In2\",\"In3\"],\"side\":\"TOP\"},\"type\":\"ConnectorPlacement.EquallySpacedRectSide\",\"uuid\":\"c52b547e-1d3f-4475-9b24-7c6221416890\"}]},\"type\":\"ConnectorPlacement.EquallySpacedConnector\",\"uuid\":\"12f77e6f-fd3f-48e5-b4f1-e7b2b8c882c1\"}],\"packageUris\":[\"http://schema.mathworks.com/mf0/Connector/R2020b\"],\"version\":\"1.0\"}"
  Quit App : Subsystem
      settings: CopyFcn=set_param(gcbh,'LinkStatus','none');
  Remove Products : Subsystem
      settings: CopyFcn=set_param(gcbh,'LinkStatus','none');  PortSchema="{\"entries\":[{\"content\":{\"sides\":[{\"content\":{},\"type\":\"ConnectorPlacement.EquallySpacedRectSide\",\"uuid\":\"bfcd81ca-6cc0-42fb-99a3-45b9e2418847\"},{\"content\":{\"side\":\"RIGHT\"},\"type\":\"ConnectorPlacement.EquallySpacedRectSide\",\"uuid\":\"2a8794f4-3879-4bca-94c5-223b002e6000\"},{\"content\":{\"connectorIds\":[\"In1\"],\"side\":\"TOP\"},\"type\":\"ConnectorPlacement.EquallySpacedRectSide\",\"uuid\":\"3a486ab2-570b-44bd-b64c-1f33147c21a8\"},{\"content\":{\"connectorIds\":[\"Out1\"],\"side\":\"BOTTOM\"},\"type\":\"ConnectorPlacement.EquallySpacedRectSide\",\"uuid\":\"938472b1-e39c-4551-af16-f13cf97987ae\"}]},\"type\":\"ConnectorPlacement.EquallySpacedConnector\",\"uuid\":\"4fcb30da-47fd-4892-8b00-93a0afe24f69\"}],\"packageUris\":[\"http://schema.mathworks.com/mf0/Connector/R2020b\"],\"version\":\"1.0\"}"
  Searching Shop / Product : Subsystem
      settings: CopyFcn=set_param(gcbh,'LinkStatus','none');  PortSchema="{\"entries\":[{\"content\":{\"sides\":[{\"content\":{},\"type\":\"ConnectorPlacement.EquallySpacedRectSide\",\"uuid\":\"bfcd81ca-6cc0-42fb-99a3-45b9e2418847\"},{\"content\":{\"side\":\"RIGHT\"},\"type\":\"ConnectorPlacement.EquallySpacedRectSide\",\"uuid\":\"2a8794f4-3879-4bca-94c5-223b002e6000\"},{\"content\":{\"connectorIds\":[\"In1\"],\"side\":\"TOP\"},\"type\":\"ConnectorPlacement.EquallySpacedRectSide\",\"uuid\":\"3a486ab2-570b-44bd-b64c-1f33147c21a8\"},{\"content\":{\"connectorIds\":[\"Out1\"],\"side\":\"BOTTOM\"},\"type\":\"ConnectorPlacement.EquallySpacedRectSide\",\"uuid\":\"eedbdb5e-dcf1-4bdd-9900-6905774af81b\"}]},\"type\":\"ConnectorPlacement.EquallySpacedConnector\",\"uuid\":\"4fcb30da-47fd-4892-8b00-93a0afe24f69\"}],\"packageUris\":[\"http://schema.mathworks.com/mf0/Connector/R2020b\"],\"version\":\"1.0\"}"
  Send Discount Notification : Subsystem
      settings: CopyFcn=set_param(gcbh,'LinkStatus','none');
  Show Invalid Login / Password : Subsystem
      settings: CopyFcn=set_param(gcbh,'LinkStatus','none');
  Show Login Successful : Subsystem
      settings: CopyFcn=set_param(gcbh,'LinkStatus','none');  PortSchema="{\"entries\":[{\"content\":{\"sides\":[{\"content\":{\"connectorIds\":[\"Out1\"]},\"type\":\"ConnectorPlacement.EquallySpacedRectSide\",\"uuid\":\"be42d590-71f1-4328-bf36-769bf487d98c\"},{\"content\":{\"connectorIds\":[\"In1\"],\"side\":\"RIGHT\"},\"type\":\"ConnectorPlacement.EquallySpacedRectSide\",\"uuid\":\"f686bdea-c754-42dd-9eaf-f93e30a31542\"},{\"content\":{\"side\":\"TOP\"},\"type\":\"ConnectorPlacement.EquallySpacedRectSide\",\"uuid\":\"aaf7fed9-1a14-44f9-b7af-ebaa0b7204d4\"},{\"content\":{\"side\":\"BOTTOM\"},\"type\":\"ConnectorPlacement.EquallySpacedRectSide\",\"uuid\":\"1006834c-f250-4b6a-aa24-ab37bbc8ba09\"}]},\"type\":\"ConnectorPlacement.EquallySpacedConnector\",\"uuid\":\"f2ca7d40-436a-4bcc-bce4-1a0ffaec5aa3\"}],\"packageUris\":[\"http://schema.mathworks.com/mf0/Connector/R2020b\"],\"version\":\"1.0\"}"
  Sign User In : Subsystem
      settings: CopyFcn=set_param(gcbh,'LinkStatus','none');  PortSchema="{\"entries\":[{\"content\":{\"sides\":[{\"content\":{},\"type\":\"ConnectorPlacement.EquallySpacedRectSide\",\"uuid\":\"873ca6fb-737d-4b52-910b-d3362c79eeee\"},{\"content\":{\"side\":\"RIGHT\"},\"type\":\"ConnectorPlacement.EquallySpacedRectSide\",\"uuid\":\"ba60fc33-b236-4c23-8fcd-c0b31457fe6e\"},{\"content\":{\"connectorIds\":[\"In1\"],\"side\":\"TOP\"},\"type\":\"ConnectorPlacement.EquallySpacedRectSide\",\"uuid\":\"e81623ee-00f7-4aa0-b91b-b5c706a16c15\"},{\"content\":{\"connectorIds\":[\"Out1\"],\"side\":\"BOTTOM\"},\"type\":\"ConnectorPlacement.EquallySpacedRectSide\",\"uuid\":\"633ed4a7-b9de-4c3c-a9f2-23ab06d69e1f\"}]},\"type\":\"ConnectorPlacement.EquallySpacedConnector\",\"uuid\":\"4a5fb8e3-3bb7-4720-ba76-c4b22f03e2da\"}],\"packageUris\":[\"http://schema.mathworks.com/mf0/Connector/R2020b\"],\"version\":\"1.0\"}"
  User Enters Account Name & Password : Subsystem
      settings: CopyFcn=set_param(gcbh,'LinkStatus','none');  PortSchema="{\"entries\":[{\"content\":{\"sides\":[{\"content\":{\"connectorIds\":[\"In1\"]},\"type\":\"ConnectorPlacement.EquallySpacedRectSide\",\"uuid\":\"3fb5762c-1463-4d69-b71f-d3478a8e66fc\"},{\"content\":{\"connectorIds\":[\"In2\",\"Out1\"],\"side\":\"RIGHT\"},\"type\":\"ConnectorPlacement.EquallySpacedRectSide\",\"uuid\":\"8c5ab484-2882-4a25-a56e-8782928f7c87\"},{\"content\":{\"side\":\"TOP\"},\"type\":\"ConnectorPlacement.EquallySpacedRectSide\",\"uuid\":\"adc29f19-0a83-4db7-81d6-093442179a8b\"}]},\"type\":\"ConnectorPlacement.EquallySpacedConnector\",\"uuid\":\"53417cf2-4b18-460a-8f45-b9110c6542e4\"}],\"packageUris\":[\"http://schema.mathworks.com/mf0/Connector/R2020b\"],\"version\":\"1.0\"}"
  View Shopping Cart : Subsystem
      settings: CopyFcn=set_param(gcbh,'LinkStatus','none');  PortSchema="{\"entries\":[{\"content\":{\"sides\":[{\"content\":{},\"type\":\"ConnectorPlacement.EquallySpacedRectSide\",\"uuid\":\"bfcd81ca-6cc0-42fb-99a3-45b9e2418847\"},{\"content\":{\"side\":\"RIGHT\"},\"type\":\"ConnectorPlacement.EquallySpacedRectSide\",\"uuid\":\"2a8794f4-3879-4bca-94c5-223b002e6000\"},{\"content\":{\"connectorIds\":[\"In1\"],\"side\":\"TOP\"},\"type\":\"ConnectorPlacement.EquallySpacedRectSide\",\"uuid\":\"3a486ab2-570b-44bd-b64c-1f33147c21a8\"},{\"content\":{\"connectorIds\":[\"Out1\"],\"side\":\"BOTTOM\"},\"type\":\"ConnectorPlacement.EquallySpacedRectSide\",\"uuid\":\"520ca31a-45cd-4e23-a10d-0a9f725daa5a\"}]},\"type\":\"ConnectorPlacement.EquallySpacedConnector\",\"uuid\":\"4fcb30da-47fd-4892-8b00-93a0afe24f69\"}],\"packageUris\":[\"http://schema.mathworks.com/mf0/Connector/R2020b\"],\"version\":\"1.0\"}"
  "[else]" : Subsystem
      settings: CopyFcn=set_param(gcbh,'LinkStatus','none');  PortSchema="{\"entries\":[{\"content\":{\"sides\":[{\"content\":{\"connectorIds\":[\"Out2\"]},\"type\":\"ConnectorPlacement.EquallySpacedRectSide\",\"uuid\":\"bfcd81ca-6cc0-42fb-99a3-45b9e2418847\"},{\"content\":{\"connectorIds\":[\"In1\",\"Out1\"],\"side\":\"RIGHT\"},\"type\":\"ConnectorPlacement.EquallySpacedRectSide\",\"uuid\":\"2a8794f4-3879-4bca-94c5-223b002e6000\"},{\"content\":{\"side\":\"TOP\"},\"type\":\"ConnectorPlacement.EquallySpacedRectSide\",\"uuid\":\"3a486ab2-570b-44bd-b64c-1f33147c21a8\"}]},\"type\":\"ConnectorPlacement.EquallySpacedConnector\",\"uuid\":\"4fcb30da-47fd-4892-8b00-93a0afe24f69\"}],\"packageUris\":[\"http://schema.mathworks.com/mf0/Connector/R2020b\"],\"version\":\"1.0\"}"
  "[else]1" : Subsystem
      settings: CopyFcn=set_param(gcbh,'LinkStatus','none');  PortSchema="{\"entries\":[{\"content\":{\"sides\":[{\"content\":{\"connectorIds\":[\"Out2\",\"In1\"]},\"type\":\"ConnectorPlacement.EquallySpacedRectSide\",\"uuid\":\"3fb5762c-1463-4d69-b71f-d3478a8e66fc\"},{\"content\":{\"connectorIds\":[\"Out1\"],\"side\":\"RIGHT\"},\"type\":\"ConnectorPlacement.EquallySpacedRectSide\",\"uuid\":\"8c5ab484-2882-4a25-a56e-8782928f7c87\"},{\"content\":{\"side\":\"TOP\"},\"type\":\"ConnectorPlacement.EquallySpacedRectSide\",\"uuid\":\"adc29f19-0a83-4db7-81d6-093442179a8b\"}]},\"type\":\"ConnectorPlacement.EquallySpacedConnector\",\"uuid\":\"53417cf2-4b18-460a-8f45-b9110c6542e4\"}],\"packageUris\":[\"http://schema.mathworks.com/mf0/Connector/R2020b\"],\"version\":\"1.0\"}"
  "[else]2" : Subsystem
      settings: CopyFcn=set_param(gcbh,'LinkStatus','none');  PortSchema="{\"entries\":[{\"content\":{\"sides\":[{\"content\":{\"connectorIds\":[\"Out2\",\"Out3\"]},\"type\":\"ConnectorPlacement.EquallySpacedRectSide\",\"uuid\":\"bfcd81ca-6cc0-42fb-99a3-45b9e2418847\"},{\"content\":{\"connectorIds\":[\"Out1\",\"In1\"],\"side\":\"RIGHT\"},\"type\":\"ConnectorPlacement.EquallySpacedRectSide\",\"uuid\":\"2a8794f4-3879-4bca-94c5-223b002e6000\"},{\"content\":{\"side\":\"TOP\"},\"type\":\"ConnectorPlacement.EquallySpacedRectSide\",\"uuid\":\"3a486ab2-570b-44bd-b64c-1f33147c21a8\"}]},\"type\":\"ConnectorPlacement.EquallySpacedConnector\",\"uuid\":\"4fcb30da-47fd-4892-8b00-93a0afe24f69\"}],\"packageUris\":[\"http://schema.mathworks.com/mf0/Connector/R2020b\"],\"version\":\"1.0\"}"
  wires:
  "[else]1"/1(Out1) -> Quit App/1(In1)
  MergeDecision1/2(Out1) -> MergeDecision2/2(In1)
  MergeDecision1/1(Out2) -> MergeDecision3/1(In1)
  MergeDecision2/1(Out1) -> Browsing Shop / Product/1(In1)
  MergeDecision3/1(Out1) -> Searching Shop / Product/1(In1)
  Browsing Shop / Product/1(Out1) -> MergeDecision4/1(In1)
  MergeDecision5/1(Out1) -> MergeDecision3/2(In2)
  MergeDecision4/2(Out1) -> MergeDecision2/1(In2)
  MergeDecision4/1(Out2) -> MergeDecision6/1(In1)
  MergeDecision5/2(Out2) -> MergeDecision6/2(In2)
  MergeDecision6/1(Out1) -> View Shopping Cart/1(In1)
  View Shopping Cart/1(Out1) -> MergeDecision7/1(In1)
  MergeDecision7/2(Out1) -> Add More Products/1(In1)
  MergeDecision7/1(Out2) -> Remove Products/1(In1)
  Add More Products/1(Out1) -> "[else]"/1(In1)
  Remove Products/1(Out1) -> MergeDecision8/1(In1)
  "[else]"/1(Out1) -> MergeDecision8/2(In2)
  "[else]"/2(Out2) -> MergeDecision1/1(In2)
  MergeDecision9/2(Out1) -> Process Online Payment Using CC / DC / Paypal  / Venmo / Alipay/1(In1)
  MergeDecision9/1(Out2) -> Process Gift Card Payment/1(In1)
  Prompt Payment Methods/1(Out1) -> MergeDecision9/1(In1)
  "[else]2"/2(Out1) -> Not Enough Money / Don't Need Product Anymore/1(In1)
  "[else]2"/3(Out2) -> Prompt Payment Methods/3(In2)
  "[else]2"/1(Out3) -> Display Review Order Interface/1(In1)
  Display Review Order Interface/1(OutputPin) -> Display Payment Confirmation Interface/1(InputPin)
  Display Delivery Information/1(OutputPin) -> Prompt GPS Tracking Function/1(InputPin)
  MergeDecision11/2(Out1) -> Collect Feedback/1(In1)
  Prompt GPS Tracking Function/1(Out1) -> MergeDecision11/1(In1)
  MergeDecision11/1(Out2) -> Order Finished/2(In1)
  MergeDecision8/1(Out1) -> JoinFork/1(In1)
  JoinFork/1(Out1) -> Prompt Discounts & Rewords/1(In1)
  JoinFork/2(Out2) -> Prompt Payment Methods/1(In1)
  Homepage/1(Out1) -> MergeDecision1/2(In1)
  Create New Merchant Account/1(OutputPin) -> Manage Merchant Account Settings/1(InputPin)
  Create New Customer Account/1(OutputPin) -> Manage Customer Account Settings/1(InputPin)
  Manage Merchant Account Settings/1(OutputPin) -> Enter / Edit Product  Menu/1(InputPin)
  MergeDecision/3(Out1) -> Enter / Edit Product Images/1(In1)
  Enter / Edit Product  Menu/1(Out1) -> MergeDecision/1(In1)
  MergeDecision/2(Out2) -> Enter / Edit Product Description/1(In1)
  MergeDecision/1(Out3) -> Enter / Edit Product  Price/1(In1)
  Enter / Edit Product  Price/1(Out1) -> MergeDecision12/2(In1)
  Enter / Edit Product Description/1(Out1) -> MergeDecision12/1(In2)
  Enter / Edit Product Images/1(Out1) -> MergeDecision12/3(In3)
  MergeDecision12/1(Out1) -> Display Login Interface/2(In2)
  Initial/1(Out1) -> Create New Customer Account/1(In1)
  Initial1/1(Out1) -> Create New Merchant Account/1(In1)
  Manage Customer Account Settings/1(OutputPin) -> Display Login Interface/1(InputPin)
  Display Login Interface/1(OutputPin) -> User Enters Account Name & Password/1(InputPin1)
  Sign User In/1(OutputPin) -> Homepage/1(InputPin)
  Display Search Result/1(Out1) -> MergeDecision5/1(In1)
  Searching Shop / Product/1(OutputPin) -> Display Search Result/1(InputPin)
  Prompt Discounts & Rewords/2(OutputPin) -> Homepage/2(InputPin1)
  Prompt Discounts & Rewords/1(OutputPin1) -> Prompt Payment Methods/2(InputPin)
  Process Online Payment Using CC / DC / Paypal  / Venmo / Alipay/1(OutputPin) -> Authenticate Payment/1(InputPin)
  Process Gift Card Payment/1(OutputPin) -> Authenticate Payment/2(InputPin1)
  Authenticate Payment/1(Out1) -> "[else]2"/1(In1)
  User Enters Account Name & Password/1(Out1) -> MergeDecision10/1(In1)
  MergeDecision10/2(Out1) -> Show Login Successful/1(In1)
  MergeDecision10/1(Out2) -> Show Invalid Login / Password/1(In2)
  Display Payment Confirmation Interface/1(OutputPin) -> Display Delivery Information/1(InputPin1)
  Collect Feedback/1(Out1) -> Order Finished/1(In2)
  Show Login Successful/1(OutputPin) -> Sign User In/1(InputPin)
  Show Invalid Login / Password/1(Out1) -> "[else]1"/1(In1)
  "[else]1"/2(Out2) -> User Enters Account Name & Password/2(In2)
  Manage Merchant Account Settings/2(OutputPin2) -> Send Discount Notification/1(InputPin)
  Manage Customer Account Settings/2(OutputPin1) -> Send Discount Notification/2(InputPin1)
  Display Review Order Interface/2(OutputPin1) -> Live Customer Support/3(InputPin2)

== system Online_Ordering_System_Activity_Diagram/Add More Products ==
  In1 : Inport
  Out1 : Outport

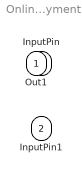
== system Online_Ordering_System_Activity_Diagram/Authenticate Payment ==
  InputPin : Inport
  InputPin1 : Inport  Port=2
  Out1 : Outport

== system Online_Ordering_System_Activity_Diagram/Browsing Shop // Product ==
  In1 : Inport
  Out1 : Outport

== system Online_Ordering_System_Activity_Diagram/Collect Feedback ==
  In1 : Inport
  Out1 : Outport

== system Online_Ordering_System_Activity_Diagram/Create New Customer Account ==
  In1 : Inport
  OutputPin : Outport  OutDataTypeStr=double  PortDimensions=1

== system Online_Ordering_System_Activity_Diagram/Create New Merchant Account ==
  In1 : Inport
  OutputPin : Outport  OutDataTypeStr=double  PortDimensions=1

== system Online_Ordering_System_Activity_Diagram/Display Delivery Information ==
  InputPin1 : Inport
  OutputPin : Outport  OutDataTypeStr=double  PortDimensions=1

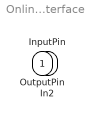
== system Online_Ordering_System_Activity_Diagram/Display Login Interface ==
  InputPin : Inport
  In2 : Inport  Port=2
  OutputPin : Outport  OutDataTypeStr=double  PortDimensions=1
